simulink model "KalmanPrep"  (R2023b)
settings: Solver=FixedStepAuto  StartTime=0.0  StopTime=20.0  FixedStep=0.001  RelTol=1e-3
values from neighbouring files (symbols this model uses):
  A = [1, Ts ... (first row only)    [KalPrep_mat.m]
  B = [Ts; 0]    [KalPrep_mat.m]
  bayas = 0.5    [KalPrep_mat.m]
  C = [1, 0]    [KalPrep_mat.m]
  cov_ic = [10, 0 ... (first row only)    [KalPrep_mat.m]    (also in Kal_6Dpitch_mat.m = cov_ic * (1 + 2*rand); Kal_pitch_mat.m = cov_ic * (1 + 2*rand))
  G = [Ts 0 ... (first row only)    [KalPrep_mat.m]    (also in Kal_6Dpitch_mat.m = eye(3) * Ts; Kal_pitch_mat.m = eye(3) * Ts)
  init_cond = [pi/2; 5]    [KalPrep_mat.m]    (also in Kal_6Dpitch_mat.m = [2; 0; 0]; Kal_pitch_mat.m = [0; 0; 0])
  K1 = 0.48    [KalPrep_mat.m]
  K2 = 0.16    [KalPrep_mat.m]
  Q = [(sig1^2), 0 ... (first row only)    [KalPrep_mat.m]    (also in Kal_6Dpitch_mat.m = zeros(3,3); Kal_pitch_mat.m = zeros(3,3))
  R = (eta1)^2    [KalPrep_mat.m]    (also in Kal_6Dpitch_mat.m = [(eta1^2), 0; Kal_pitch_mat.m = [eta1, 0; untitled.m = 10)
libraries: dspsrcs4 x2
settings Model: Creator=fabio  LastModifiedBy=fabio

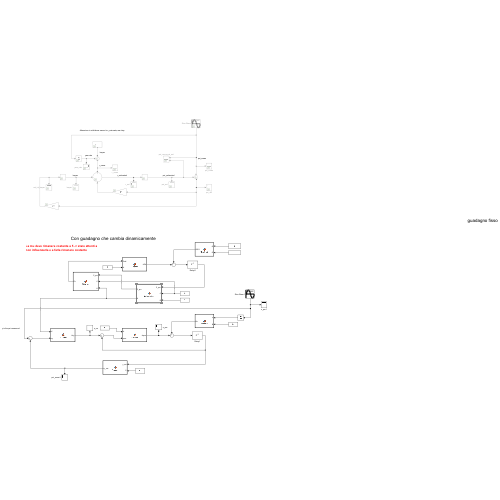
[thumbnail: Simulink's stored preview of the top-level diagram]
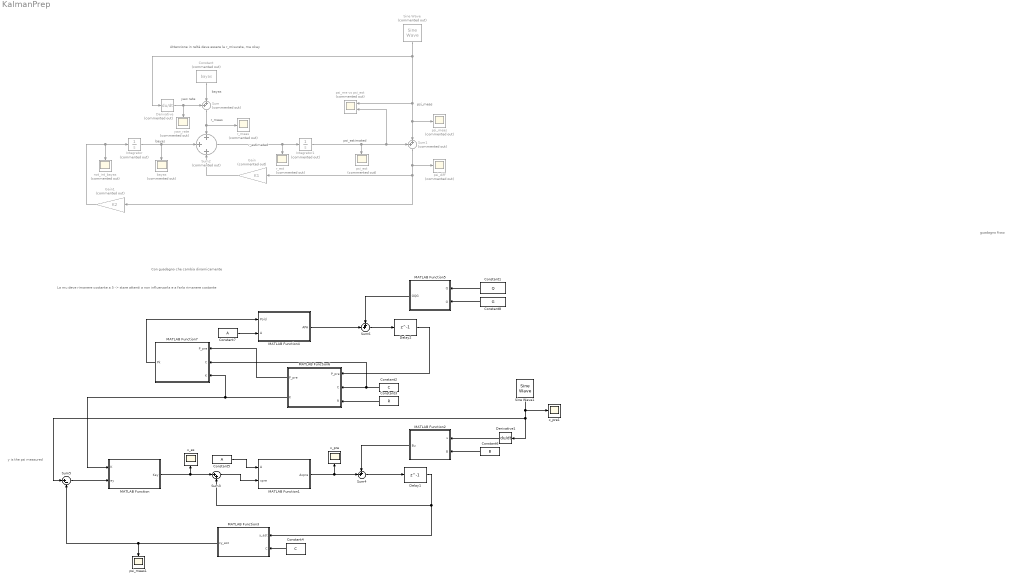
== system KalmanPrep ==
  note: La mu deve rimanere costante a 5 -> stare attenti a non influenzarla e a farla rimanere costante
  note: guadagno fisso
  note: Con guadagno che cambia dinamicamente
  note: y is the psi measured
  note: Attenzione in reltà deve essere la r_misurata, ma okay
  note: psi_meas
  note: yaw rate
  note: bayas
  note: r_meas
  note: bayas
  note: r_estimated
  note: psi_estimated
  Constant : Constant  Commented=on  Value=bayas
  Constant1 : Constant  Value=Q
  Constant2 : Constant  Value=C  VectorParams1D=off
  Constant3 : Constant  Value=R
  Constant4 : Constant  Value=C  VectorParams1D=off
  Constant5 : Constant  Value=A
  Constant6 : Constant  Value=B
  Constant7 : Constant  Value=A
  Constant8 : Constant  Value=G
  Delay1 : Delay  DelayLength=1  InitialCondition=init_cond  UseCircularBuffer=on
  Delay2 : Delay  DelayLength=1  InitialCondition=cov_ic  UseCircularBuffer=on
  Derivative : Derivative  Commented=on
  Derivative1 : Derivative
  Gain : Gain  Commented=on  Gain=K1
  Gain1 : Gain  Commented=on  Gain=K2
  Integrator : Integrator  Commented=on
  Integrator1 : Integrator  Commented=on
  MATLAB Function : MATLAB Function  TreatAsAtomicUnit=on
  MATLAB Function1 : MATLAB Function  TreatAsAtomicUnit=on
  MATLAB Function2 : MATLAB Function  TreatAsAtomicUnit=on
  MATLAB Function3 : MATLAB Function  TreatAsAtomicUnit=on
  MATLAB Function4 : MATLAB Function  TreatAsAtomicUnit=on
  MATLAB Function5 : MATLAB Function  TreatAsAtomicUnit=on
  MATLAB Function6 : MATLAB Function  TreatAsAtomicUnit=on
  MATLAB Function7 : MATLAB Function  TreatAsAtomicUnit=on
  Sine Wave : dspsrcs4/Sine Wave  Commented=on  Amplitude=1  Frequency=100  Phase=0  SampleMode=Discrete  OutComplex=Real  CompMethod=Trigonometric fcn  TableSize=Speed  SampleTime=1/1000  SamplesPerFrame=1  ResetState=Restart at time zero  OutputFrames=off  dataType=double  wordLen=16  udDataType=sfix(16)  fracBitsMode=Best precision  numFracBits=15  OutDataTypeStr=double  LastOutDataTypeStr=double
  Sine Wave1 : dspsrcs4/Sine Wave  Amplitude=1  Frequency=100  Phase=0  SampleMode=Discrete  OutComplex=Real  CompMethod=Trigonometric fcn  TableSize=Speed  SampleTime=1/1000  SamplesPerFrame=1  ResetState=Restart at time zero  OutputFrames=off  dataType=double  wordLen=16  udDataType=sfix(16)  fracBitsMode=Best precision  numFracBits=15  OutDataTypeStr=double  LastOutDataTypeStr=double
  Sum : Sum  Commented=on  Inputs=++|
  Sum1 : Sum  Commented=on  Inputs=++|
  Sum2 : Sum  Commented=on  Inputs=+||+||+
  Sum3 : Sum  Inputs=|++
  Sum4 : Sum  Inputs=++|
  Sum5 : Sum  Inputs=|+-
  Sum6 : Sum  Inputs=++|
  bayas : Scope  Commented=on
  not_int_bayas : Scope  Commented=on
  psi_diff : Scope  Commented=on
  psi_est : Scope  Commented=on
  psi_me vs psi_est : Scope  Commented=on  NumInputPorts=2
  psi_meas : Scope  Commented=on
  psi_meas1 : Scope
  r_est : Scope  Commented=on
  r_meas : Scope  Commented=on
  x_es : Scope
  x_pre : Scope
  x_pre1 : Scope
  yaw_rate : Scope  Commented=on
  wires:
  Derivative/1 -> yaw_rate/1, Sum/1
  Constant/1 -> Sum/2
  Sine Wave/1 -> Derivative/1, Sum1/2, psi_meas/1, psi_me vs psi_est/1
  Sum/1 -> Sum2/1, r_meas/1
  Integrator/1 -> Sum2/2, bayas/1
  Sum2/1 -> r_est/1, Integrator1/1
  Integrator1/1 -> psi_est/1, psi_me vs psi_est/2, Sum1/1
  Gain/1 -> Sum2/3
  Sum1/1 -> psi_diff/1, Gain1/1, Gain/1
  Gain1/1 -> not_int_bayas/1, Integrator/1
  MATLAB Function/1(Key) -> x_es/1, Sum3/1
  Sum3/1 -> MATLAB Function1/2(xpre)
  MATLAB Function1/1(Axpre) -> x_pre/1, Sum4/2
  MATLAB Function2/1(Bu) -> Sum4/1
  Sum4/1 -> Delay1/1
  Delay1/1 -> Sum3/2, MATLAB Function3/1(y_est)
  Sum5/1 -> MATLAB Function/2(ey)
  MATLAB Function3/1(cy_est) -> Sum5/2, psi_meas1/1
  MATLAB Function5/1(GQG) -> Sum6/1
  MATLAB Function4/1(APA) -> Sum6/2
  Delay2/1 -> MATLAB Function6/1("P_pre ")
  Sum6/1 -> Delay2/1
  Constant1/1 -> MATLAB Function5/1(Q)
  MATLAB Function6/2(K) -> MATLAB Function7/3(K), MATLAB Function/1(K)
  Constant2/1 -> MATLAB Function7/2(C), MATLAB Function6/2(C)
  Constant3/1 -> MATLAB Function6/3(R)
  MATLAB Function7/1(Pk) -> MATLAB Function4/1(Pold)
  Constant4/1 -> MATLAB Function3/2(C)
  Sine Wave1/1 -> Sum5/1, Derivative1/1, x_pre1/1
  Constant5/1 -> MATLAB Function1/1(A)
  Constant6/1 -> MATLAB Function2/2(B)
  Constant7/1 -> MATLAB Function4/2(A)
  Constant8/1 -> MATLAB Function5/2(G)
  MATLAB Function6/1(P_pre) -> MATLAB Function7/1(P_pre)
  Derivative1/1 -> MATLAB Function2/1(u)

== matlab function KalmanPrep/MATLAB Function1 ==
  data: A input; xpre input; Axpre output
function Axpre= Amatrix(A, xpre)
    Axpre = A * xpre;

== matlab function KalmanPrep/MATLAB Function ==
  data: K input; ey input; Key output
function Key = GainMult(K, ey)
    Key = K*ey; % 2x1

== matlab function KalmanPrep/MATLAB Function2 ==
  data: u input; Bu output; B input
function Bu = Bmatrix(u, B) 
    Bu = B * u;

== matlab function KalmanPrep/MATLAB Function3 ==
  data: y_est input; cy_est output; C input
function cy_est = Cmatrix(y_est, C)
    cy_est = C * y_est; % 1x1

== matlab function KalmanPrep/MATLAB Function4 ==
  data: Pold input; APA output; A input
function APA = Amatrix(Pold, A)
    APA = A*Pold*(A');

== matlab function KalmanPrep/MATLAB Function5 ==
  data: Q input; GQG output; G input
function GQG = GmatrixQ(Q, G)
    GQG = G*Q*(G');

== matlab function KalmanPrep/MATLAB Function6 ==
  data: P_pre output; P_pre input; C input; K output; R input
function [P_pre, K] = KalmanGain(P_pre, C, R)
    K = zeros(2,1);
    K = (P_pre*(C'))*pinv((C*P_pre*(C') + R)); % 2x1

== matlab function KalmanPrep/MATLAB Function7 ==
  data: P_pre input; C input; Pk output; K input
function Pk = PkComp(P_pre, C, K)
    I = eye(2); % mod con dimesnione K*C
    Pk = (I - K*C)*P_pre; % 2x2 ok
